simulink model "copper_solvent_extraction_model_simulink"  (R2021a)
settings: Solver=ode14x  StartTime=0.0  StopTime=simulation_time  FixedStep=step_time  RelTol=1e-3
undefined symbols (not defined in the file): C1_aq_ss, C1_el_ss, C1_org_ss, C2_aq_ss, C2_org_ss, C3_aq_ss, C3_org_ss, C4_org_ss, C_aq_max, C_org_max, cLE_ss, cPLS_ss, EXTERNAL_VARIABLES_STEADY_STATE, fLE_max, fLO_max, fPLSP_ss, fPLSS_ss, I_FB1, I_FB2, K_eq_ext, K_eq_str, K_ff_FF1, K_ff_FF2, K_ff_FF3, K_ff_FF4, K_mass_1, K_mass_2, K_mass_3, K_mass_4, Kb_FB1, Kb_FB2, Kc_FB1, Kc_FB2, LOWPASS_FILTER_TUNING, seed_c_BO, seed_c_LE, seed_c_LO, seed_c_PLS, seed_c_RaffP, seed_c_RaffS, seed_c_RE, seed_f_LE, seed_f_LO, seed_f_PLSP, seed_f_PLSS, sigma_c_BO, sigma_c_LE, sigma_c_LO, sigma_c_PLS, sigma_c_RaffP, sigma_c_RaffS, sigma_c_RE, sigma_f_LE, sigma_f_LO, sigma_f_PLSP, sigma_f_PLSS, step_time, t1, t2, t3 ... (+43)
libraries: cstblocks x4, pid_lib x2
(part 1 of 3)
settings Model: Creator=piete  LastModifiedBy=piete
settings DataIOCC: ReturnWorkspaceOutputsName=simulation_results

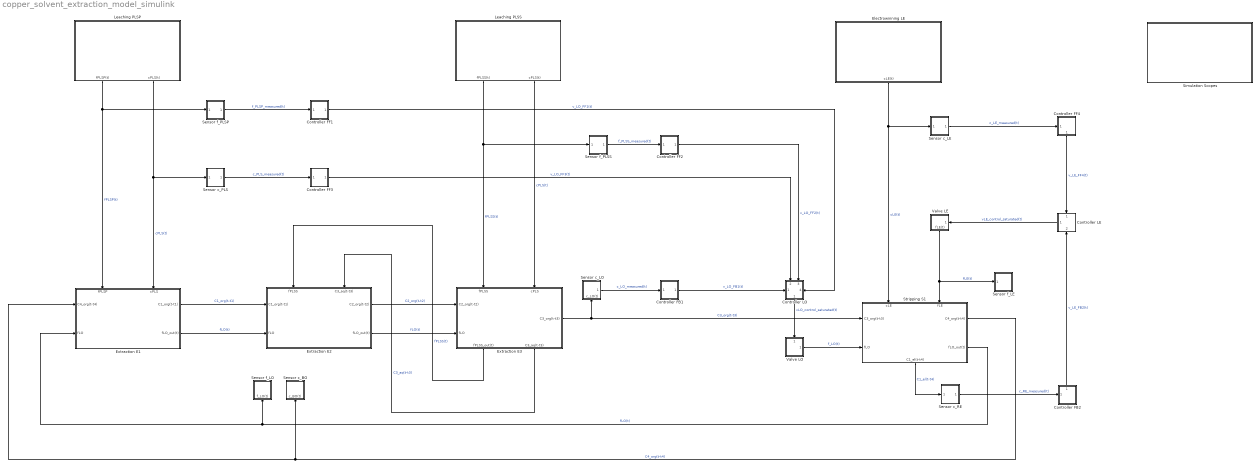
== system copper_solvent_extraction_model_simulink ==
  "                           Controller LO" : Subsystem
      settings: PortSchema="{\"entries\":[{\"content\":{\"sides\":[{\"content\":{\"connectorIds\":[\"In1\"]},\"type\":\"ConnectorPlacement.EquallySpacedRectSide\",\"uuid\":\"52743177-f082-4040-b095-38ff8f699919\"},{\"content\":{\"connectorIds\":[\"In4\"],\"side\":\"RIGHT\"},\"type\":\"ConnectorPlacement.EquallySpacedRectSide\",\"uuid\":\"070049ef-ea19-4899-84de-48e128addf57\"},{\"content\":{\"connectorIds\":[\"In2\",\"In3\"],\"side\":\"TOP\"},\"type\":\"ConnectorPlacement.EquallySpacedRectSide\",\"uuid\":\"35f470f2-3d73-4a31-9332-3265bce356f1\"},{\"content\":{\"connectorIds\":[\"Out1\"],\"side\":\"BOTTOM\"},\"type\":\"ConnectorPlacement.EquallySpacedRectSide\",\"uuid\":\"171e56ae-489a-47d3-90fa-98f8654578fe\"}]},\"type\":\"ConnectorPlacement.EquallySpacedConnector\",\"uuid\":\"0a01319a-d0cf-448a-a915-1b81fd6ea2a4\"}],\"packageUris\":[\"http://schema.mathworks.com/mf0/Connector/R2020b\"],\"version\":\"1.0\"}"
      mask Display: image('.\assets\simulink\controllers\c_LO_controller.png'); % Use "Edit Image" on toolstrip to change.
  Controller FB1 : Subsystem
      mask Display: image('.\assets\simulink\controllers\controller_FB1.png'); % Use "Edit Image" on toolstrip to change.
  Controller FB2 : Subsystem
      settings: PortSchema="{\"entries\":[{\"content\":{\"sides\":[{\"content\":{\"connectorIds\":[\"In1\"]},\"type\":\"ConnectorPlacement.EquallySpacedRectSide\",\"uuid\":\"549d450d-0da5-494d-9dce-c33c7378f634\"},{\"content\":{\"connectorIds\":[],\"side\":\"RIGHT\"},\"type\":\"ConnectorPlacement.EquallySpacedRectSide\",\"uuid\":\"cc4f927b-a34a-449e-b64f-caed187c260d\"},{\"content\":{\"connectorIds\":[\"Out1\"],\"side\":\"TOP\"},\"type\":\"ConnectorPlacement.EquallySpacedRectSide\",\"uuid\":\"b52d82b8-907a-4fce-9f5e-46f0b202510f\"}]},\"type\":\"ConnectorPlacement.EquallySpacedConnector\",\"uuid\":\"8987fc10-9638-4425-b9e3-d065bbee564b\"}],\"packageUris\":[\"http://schema.mathworks.com/mf0/Connector/R2020b\"],\"version\":\"1.0\"}"
      mask Display: image('.\assets\simulink\controllers\controller_FB2.png'); % Use "Edit Image" on toolstrip to change.
  Controller FF1 : Subsystem
      mask Display: image('.\assets\simulink\controllers\controller_FF1.png'); % Use "Edit Image" on toolstrip to change.
  Controller FF2 : Subsystem
      mask Display: image('.\assets\simulink\controllers\controller_FF2.png'); % Use "Edit Image" on toolstrip to change.
  Controller FF3 : Subsystem
      mask Display: image('.\assets\simulink\controllers\controller_FF3.png'); % Use "Edit Image" on toolstrip to change.
  Controller FF4 : Subsystem
      settings: PortSchema="{\"entries\":[{\"content\":{\"sides\":[{\"content\":{\"connectorIds\":[\"In1\"]},\"type\":\"ConnectorPlacement.EquallySpacedRectSide\",\"uuid\":\"309a0a3d-e30b-4a77-b5d2-c4b50080f33a\"},{\"content\":{\"connectorIds\":[],\"side\":\"RIGHT\"},\"type\":\"ConnectorPlacement.EquallySpacedRectSide\",\"uuid\":\"b344a8f7-ad8f-4273-abc7-1e7d20895348\"},{\"content\":{\"connectorIds\":[],\"side\":\"TOP\"},\"type\":\"ConnectorPlacement.EquallySpacedRectSide\",\"uuid\":\"47acaef9-06fd-4941-bd8f-4f44734e5892\"},{\"content\":{\"connectorIds\":[\"Out1\"],\"side\":\"BOTTOM\"},\"type\":\"ConnectorPlacement.EquallySpacedRectSide\",\"uuid\":\"0fe3c328-0dcb-42fe-b977-ff04426d3ff8\"}]},\"type\":\"ConnectorPlacement.EquallySpacedConnector\",\"uuid\":\"cf890694-841f-4aa2-8bc3-028381901d63\"}],\"packageUris\":[\"http://schema.mathworks.com/mf0/Connector/R2020b\"],\"version\":\"1.0\"}"
      mask Display: image('.\assets\simulink\controllers\controller_FF4.png'); % Use "Edit Image" on toolstrip to change.
  Controller LE : Subsystem
      settings: PortSchema="{\"entries\":[{\"content\":{\"sides\":[{\"content\":{\"connectorIds\":[]},\"type\":\"ConnectorPlacement.EquallySpacedRectSide\",\"uuid\":\"549d450d-0da5-494d-9dce-c33c7378f634\"},{\"content\":{\"connectorIds\":[\"Out1\"],\"side\":\"RIGHT\"},\"type\":\"ConnectorPlacement.EquallySpacedRectSide\",\"uuid\":\"cc4f927b-a34a-449e-b64f-caed187c260d\"},{\"content\":{\"connectorIds\":[\"In1\"],\"side\":\"TOP\"},\"type\":\"ConnectorPlacement.EquallySpacedRectSide\",\"uuid\":\"b52d82b8-907a-4fce-9f5e-46f0b202510f\"},{\"content\":{\"connectorIds\":[\"In2\"],\"side\":\"BOTTOM\"},\"type\":\"ConnectorPlacement.EquallySpacedRectSide\",\"uuid\":\"d43d3a57-d85d-4e24-871d-d5e185b00129\"}]},\"type\":\"ConnectorPlacement.EquallySpacedConnector\",\"uuid\":\"8987fc10-9638-4425-b9e3-d065bbee564b\"}],\"packageUris\":[\"http://schema.mathworks.com/mf0/Connector/R2020b\"],\"version\":\"1.0\"}"
      mask Display: image('.\assets\simulink\controllers\c_RE_controller.png'); % Use "Edit Image" on toolstrip to change.
  Electrowinning LE : Subsystem
      settings: PortSchema="{\"entries\":[{\"content\":{\"sides\":[{\"content\":{\"connectorIds\":[]},\"type\":\"ConnectorPlacement.EquallySpacedRectSide\",\"uuid\":\"d08e9f48-9437-4d33-afd1-67836a5fb6bd\"},{\"content\":{\"connectorIds\":[],\"side\":\"RIGHT\"},\"type\":\"ConnectorPlacement.EquallySpacedRectSide\",\"uuid\":\"a0c0d898-7ac9-474d-9070-540f9b51cc10\"},{\"content\":{\"connectorIds\":[],\"side\":\"TOP\"},\"type\":\"ConnectorPlacement.EquallySpacedRectSide\",\"uuid\":\"8a168008-9249-431e-9938-add887b6cc49\"},{\"content\":{\"connectorIds\":[\"Out1\"],\"side\":\"BOTTOM\"},\"type\":\"ConnectorPlacement.EquallySpacedRectSide\",\"uuid\":\"b6c2cc53-6d77-4314-bf25-d5a8095a8509\"}]},\"type\":\"ConnectorPlacement.EquallySpacedConnector\",\"uuid\":\"c94c7a5d-e9b9-4155-acb9-8888f4595dcb\"}],\"packageUris\":[\"http://schema.mathworks.com/mf0/Connector/R2020b\"],\"version\":\"1.0\"}"
      mask Display: image('.\assets\simulink\main_processes\LE.png'); % Use "Edit Image" on toolstrip to change.
  Extraction E1 : Subsystem
      settings: PortSchema="{\"entries\":[{\"content\":{\"sides\":[{\"content\":{\"connectorIds\":[\"In1\",\"In2\"]},\"type\":\"ConnectorPlacement.EquallySpacedRectSide\",\"uuid\":\"f32559ae-5e45-417b-8c50-adbeea9a29f4\"},{\"content\":{\"connectorIds\":[\"Out1\",\"Out2\"],\"side\":\"RIGHT\"},\"type\":\"ConnectorPlacement.EquallySpacedRectSide\",\"uuid\":\"22bc39ae-803b-4947-b021-a54bd767cf3b\"},{\"content\":{\"connectorIds\":[\"In3\",\"In4\"],\"side\":\"TOP\"},\"type\":\"ConnectorPlacement.EquallySpacedRectSide\",\"uuid\":\"d59dc34f-8db0-4177-a2fb-6760d02603f2\"}]},\"type\":\"ConnectorPlacement.EquallySpacedConnector\",\"uuid\":\"eadb17fe-3c9c-4f7d-9ae7-0fe299ce1ce3\"}],\"packageUris\":[\"http://schema.mathworks.com/mf0/Connector/R2020b\"],\"version\":\"1.0\"}"
      mask Display: image('.\assets\simulink\main_processes\E1.png'); % Use "Edit Image" on toolstrip to change.
  Extraction E2 : Subsystem
      settings: PortSchema="{\"entries\":[{\"content\":{\"sides\":[{\"content\":{\"connectorIds\":[\"In1\",\"In2\"]},\"type\":\"ConnectorPlacement.EquallySpacedRectSide\",\"uuid\":\"f32559ae-5e45-417b-8c50-adbeea9a29f4\"},{\"content\":{\"connectorIds\":[\"Out1\",\"Out2\"],\"side\":\"RIGHT\"},\"type\":\"ConnectorPlacement.EquallySpacedRectSide\",\"uuid\":\"22bc39ae-803b-4947-b021-a54bd767cf3b\"},{\"content\":{\"connectorIds\":[\"In3\",\"In4\"],\"side\":\"TOP\"},\"type\":\"ConnectorPlacement.EquallySpacedRectSide\",\"uuid\":\"d59dc34f-8db0-4177-a2fb-6760d02603f2\"}]},\"type\":\"ConnectorPlacement.EquallySpacedConnector\",\"uuid\":\"eadb17fe-3c9c-4f7d-9ae7-0fe299ce1ce3\"}],\"packageUris\":[\"http://schema.mathworks.com/mf0/Connector/R2020b\"],\"version\":\"1.0\"}"
      mask Display: image('.\assets\simulink\main_processes\E2.png'); % Use "Edit Image" on toolstrip to change.
  Extraction E3 : Subsystem
      settings: PortSchema="{\"entries\":[{\"content\":{\"sides\":[{\"content\":{\"connectorIds\":[\"In1\",\"In2\"]},\"type\":\"ConnectorPlacement.EquallySpacedRectSide\",\"uuid\":\"f32559ae-5e45-417b-8c50-adbeea9a29f4\"},{\"content\":{\"connectorIds\":[\"Out1\"],\"side\":\"RIGHT\"},\"type\":\"ConnectorPlacement.EquallySpacedRectSide\",\"uuid\":\"22bc39ae-803b-4947-b021-a54bd767cf3b\"},{\"content\":{\"connectorIds\":[\"In3\",\"In4\"],\"side\":\"TOP\"},\"type\":\"ConnectorPlacement.EquallySpacedRectSide\",\"uuid\":\"d59dc34f-8db0-4177-a2fb-6760d02603f2\"},{\"content\":{\"connectorIds\":[\"Out2\",\"Out3\"],\"side\":\"BOTTOM\"},\"type\":\"ConnectorPlacement.EquallySpacedRectSide\",\"uuid\":\"fbeb4835-7edf-4107-b431-1a8f0a3c5582\"}]},\"type\":\"ConnectorPlacement.EquallySpacedConnector\",\"uuid\":\"eadb17fe-3c9c-4f7d-9ae7-0fe299ce1ce3\"}],\"packageUris\":[\"http://schema.mathworks.com/mf0/Connector/R2020b\"],\"version\":\"1.0\"}"
      mask Display: image('.\assets\simulink\main_processes\E3.png'); % Use "Edit Image" on toolstrip to change.
  Leaching PLSP : Subsystem
      settings: PortSchema="{\"entries\":[{\"content\":{\"sides\":[{\"content\":{\"connectorIds\":[]},\"type\":\"ConnectorPlacement.EquallySpacedRectSide\",\"uuid\":\"350927fc-4dd2-494c-92db-8910e4459de4\"},{\"content\":{\"connectorIds\":[],\"side\":\"RIGHT\"},\"type\":\"ConnectorPlacement.EquallySpacedRectSide\",\"uuid\":\"54b31e5b-e75a-43e6-8723-66b6669f42f1\"},{\"content\":{\"connectorIds\":[],\"side\":\"TOP\"},\"type\":\"ConnectorPlacement.EquallySpacedRectSide\",\"uuid\":\"70d3a06c-9c50-446d-baab-5ad4a4ca1d21\"},{\"content\":{\"connectorIds\":[\"Out1\",\"Out2\"],\"side\":\"BOTTOM\"},\"type\":\"ConnectorPlacement.EquallySpacedRectSide\",\"uuid\":\"692c27e6-c427-4995-97d0-ac5f1bf9d541\"}]},\"type\":\"ConnectorPlacement.EquallySpacedConnector\",\"uuid\":\"478cabe5-44a5-4e19-b357-ea716b81ddf8\"}],\"packageUris\":[\"http://schema.mathworks.com/mf0/Connector/R2020b\"],\"version\":\"1.0\"}"
      mask Display: image('.\assets\simulink\main_processes\PLSP.png'); % Use "Edit Image" on toolstrip to change.
  Leaching PLSS : Subsystem
      settings: PortSchema="{\"entries\":[{\"content\":{\"sides\":[{\"content\":{\"connectorIds\":[]},\"type\":\"ConnectorPlacement.EquallySpacedRectSide\",\"uuid\":\"350927fc-4dd2-494c-92db-8910e4459de4\"},{\"content\":{\"connectorIds\":[],\"side\":\"RIGHT\"},\"type\":\"ConnectorPlacement.EquallySpacedRectSide\",\"uuid\":\"54b31e5b-e75a-43e6-8723-66b6669f42f1\"},{\"content\":{\"connectorIds\":[],\"side\":\"TOP\"},\"type\":\"ConnectorPlacement.EquallySpacedRectSide\",\"uuid\":\"70d3a06c-9c50-446d-baab-5ad4a4ca1d21\"},{\"content\":{\"connectorIds\":[\"Out1\",\"Out2\"],\"side\":\"BOTTOM\"},\"type\":\"ConnectorPlacement.EquallySpacedRectSide\",\"uuid\":\"692c27e6-c427-4995-97d0-ac5f1bf9d541\"}]},\"type\":\"ConnectorPlacement.EquallySpacedConnector\",\"uuid\":\"478cabe5-44a5-4e19-b357-ea716b81ddf8\"}],\"packageUris\":[\"http://schema.mathworks.com/mf0/Connector/R2020b\"],\"version\":\"1.0\"}"
      mask Display: image('.\assets\simulink\main_processes\PLSS.png'); % Use "Edit Image" on toolstrip to change.
  Sensor c_BO : Subsystem
      settings: PortSchema="{\"entries\":[{\"content\":{\"sides\":[{\"content\":{\"connectorIds\":[]},\"type\":\"ConnectorPlacement.EquallySpacedRectSide\",\"uuid\":\"6f225f75-77bd-4d33-9eaa-68626f4c93f8\"},{\"content\":{\"connectorIds\":[],\"side\":\"RIGHT\"},\"type\":\"ConnectorPlacement.EquallySpacedRectSide\",\"uuid\":\"fc49b7bf-677f-4e67-b426-d7f20682fd5b\"},{\"content\":{\"connectorIds\":[],\"side\":\"TOP\"},\"type\":\"ConnectorPlacement.EquallySpacedRectSide\",\"uuid\":\"0f66abcc-726d-4049-9a2a-f7387bb5b454\"},{\"content\":{\"connectorIds\":[\"In1\"],\"side\":\"BOTTOM\"},\"type\":\"ConnectorPlacement.EquallySpacedRectSide\",\"uuid\":\"02c1b306-9984-45d6-a119-b92d8916e7f3\"}]},\"type\":\"ConnectorPlacement.EquallySpacedConnector\",\"uuid\":\"3246ee4f-c332-4bf0-a096-1d04253049f7\"}],\"packageUris\":[\"http://schema.mathworks.com/mf0/Connector/R2020b\"],\"version\":\"1.0\"}"
      mask Display: image('.\assets\simulink\sensors\c_BO_sensor.png'); % Use "Edit Image" on toolstrip to change.
  Sensor c_LE : Subsystem
      mask Display: image('.\assets\simulink\sensors\c_LE_sensor.png'); % Use "Edit Image" on toolstrip to change.
  Sensor c_LO : Subsystem
      settings: PortSchema="{\"entries\":[{\"content\":{\"sides\":[{\"content\":{\"connectorIds\":[]},\"type\":\"ConnectorPlacement.EquallySpacedRectSide\",\"uuid\":\"6f225f75-77bd-4d33-9eaa-68626f4c93f8\"},{\"content\":{\"connectorIds\":[\"Out1\"],\"side\":\"RIGHT\"},\"type\":\"ConnectorPlacement.EquallySpacedRectSide\",\"uuid\":\"fc49b7bf-677f-4e67-b426-d7f20682fd5b\"},{\"content\":{\"connectorIds\":[],\"side\":\"TOP\"},\"type\":\"ConnectorPlacement.EquallySpacedRectSide\",\"uuid\":\"0f66abcc-726d-4049-9a2a-f7387bb5b454\"},{\"content\":{\"connectorIds\":[\"In1\"],\"side\":\"BOTTOM\"},\"type\":\"ConnectorPlacement.EquallySpacedRectSide\",\"uuid\":\"02c1b306-9984-45d6-a119-b92d8916e7f3\"}]},\"type\":\"ConnectorPlacement.EquallySpacedConnector\",\"uuid\":\"3246ee4f-c332-4bf0-a096-1d04253049f7\"}],\"packageUris\":[\"http://schema.mathworks.com/mf0/Connector/R2020b\"],\"version\":\"1.0\"}"
      mask Display: image('.\assets\simulink\sensors\c_LO_sensor.png'); % Use "Edit Image" on toolstrip to change.
  Sensor c_PLS : Subsystem
      mask Display: image('.\assets\simulink\sensors\c_PLS_sensor.png'); % Use "Edit Image" on toolstrip to change.
  Sensor c_RE : Subsystem
      mask Display: image('.\assets\simulink\sensors\c_RE_sensor.png'); % Use "Edit Image" on toolstrip to change.
  Sensor f_LE : Subsystem
      mask Display: image('.\assets\simulink\sensors\f_LE_sensor.png'); % Use "Edit Image" on toolstrip to change.
  Sensor f_LO : Subsystem
      settings: PortSchema="{\"entries\":[{\"content\":{\"sides\":[{\"content\":{\"connectorIds\":[]},\"type\":\"ConnectorPlacement.EquallySpacedRectSide\",\"uuid\":\"6f225f75-77bd-4d33-9eaa-68626f4c93f8\"},{\"content\":{\"connectorIds\":[],\"side\":\"RIGHT\"},\"type\":\"ConnectorPlacement.EquallySpacedRectSide\",\"uuid\":\"fc49b7bf-677f-4e67-b426-d7f20682fd5b\"},{\"content\":{\"connectorIds\":[],\"side\":\"TOP\"},\"type\":\"ConnectorPlacement.EquallySpacedRectSide\",\"uuid\":\"0f66abcc-726d-4049-9a2a-f7387bb5b454\"},{\"content\":{\"connectorIds\":[\"In1\"],\"side\":\"BOTTOM\"},\"type\":\"ConnectorPlacement.EquallySpacedRectSide\",\"uuid\":\"9f64ef61-0078-4c2b-bb4e-a94dd0622467\"}]},\"type\":\"ConnectorPlacement.EquallySpacedConnector\",\"uuid\":\"3246ee4f-c332-4bf0-a096-1d04253049f7\"}],\"packageUris\":[\"http://schema.mathworks.com/mf0/Connector/R2020b\"],\"version\":\"1.0\"}"
      mask Display: image('.\assets\simulink\sensors\f_LO_sensor.png'); % Use "Edit Image" on toolstrip to change.
  Sensor f_PLSP : Subsystem
      mask Display: image('.\assets\simulink\sensors\f_PLSP_sensor.png'); % Use "Edit Image" on toolstrip to change.
  Sensor f_PLSS : Subsystem
      mask Display: image('.\assets\simulink\sensors\f_PLSS_sensor.png'); % Use "Edit Image" on toolstrip to change.
  Simulation Scopes : Subsystem
      mask Display: image('.\assets\simulink\main_processes\scopes.png'); % Use "Edit Image" on toolstrip to change.
  Stripping S1 : Subsystem
      settings: PortSchema="{\"entries\":[{\"content\":{\"sides\":[{\"content\":{\"connectorIds\":[\"In1\",\"In2\"]},\"type\":\"ConnectorPlacement.EquallySpacedRectSide\",\"uuid\":\"edd2b024-3361-40c1-bf48-03bacc8752ae\"},{\"content\":{\"connectorIds\":[\"Out1\",\"Out2\"],\"side\":\"RIGHT\"},\"type\":\"ConnectorPlacement.EquallySpacedRectSide\",\"uuid\":\"73229bfa-5f94-46f0-92ab-46840454d51f\"},{\"content\":{\"connectorIds\":[\"In3\",\"In4\"],\"side\":\"TOP\"},\"type\":\"ConnectorPlacement.EquallySpacedRectSide\",\"uuid\":\"93068968-7869-4ed0-814c-03a88b1ad5d7\"},{\"content\":{\"connectorIds\":[\"Out3\"],\"side\":\"BOTTOM\"},\"type\":\"ConnectorPlacement.EquallySpacedRectSide\",\"uuid\":\"05c22c48-5ee0-4944-946b-00d184f09bd6\"}]},\"type\":\"ConnectorPlacement.EquallySpacedConnector\",\"uuid\":\"bf2ed9fb-a5ec-4d53-b289-eba7aea4b2cc\"}],\"packageUris\":[\"http://schema.mathworks.com/mf0/Connector/R2020b\"],\"version\":\"1.0\"}"
      mask Display: image('.\assets\simulink\main_processes\S1.png'); % Use "Edit Image" on toolstrip to change.
  Valve LE : Subsystem
      settings: PortSchema="{\"entries\":[{\"content\":{\"sides\":[{\"content\":{\"connectorIds\":[\"In1\"]},\"type\":\"ConnectorPlacement.EquallySpacedRectSide\",\"uuid\":\"06bfa01a-e663-49ea-90bb-597467147bdb\"},{\"content\":{\"connectorIds\":[],\"side\":\"RIGHT\"},\"type\":\"ConnectorPlacement.EquallySpacedRectSide\",\"uuid\":\"1b97bf0a-d157-483d-9143-b19205f93668\"},{\"content\":{\"connectorIds\":[],\"side\":\"TOP\"},\"type\":\"ConnectorPlacement.EquallySpacedRectSide\",\"uuid\":\"96bb4535-0a27-4f39-8065-f058199dbb07\"},{\"content\":{\"connectorIds\":[\"Out1\"],\"side\":\"BOTTOM\"},\"type\":\"ConnectorPlacement.EquallySpacedRectSide\",\"uuid\":\"185cf173-893e-45df-b22c-8330d77439f7\"}]},\"type\":\"ConnectorPlacement.EquallySpacedConnector\",\"uuid\":\"e8ce835b-977e-44e0-89a4-4c36a3371ef1\"}],\"packageUris\":[\"http://schema.mathworks.com/mf0/Connector/R2020b\"],\"version\":\"1.0\"}"
      mask Display: image('.\assets\simulink\valves\Valve_LE.png'); % Use "Edit Image" on toolstrip to change.
  Valve LO : Subsystem
      settings: PortSchema="{\"entries\":[{\"content\":{\"sides\":[{\"content\":{\"connectorIds\":[]},\"type\":\"ConnectorPlacement.EquallySpacedRectSide\",\"uuid\":\"6fe3adae-c1d5-49c5-9f64-d9648a674ed6\"},{\"content\":{\"connectorIds\":[\"Out1\"],\"side\":\"RIGHT\"},\"type\":\"ConnectorPlacement.EquallySpacedRectSide\",\"uuid\":\"5144e458-c494-45ed-932f-5f38aa1be950\"},{\"content\":{\"connectorIds\":[\"In1\"],\"side\":\"TOP\"},\"type\":\"ConnectorPlacement.EquallySpacedRectSide\",\"uuid\":\"1ebd3b40-fd5b-41a9-a787-94161d466247\"}]},\"type\":\"ConnectorPlacement.EquallySpacedConnector\",\"uuid\":\"aaf376a4-907c-4b9b-913e-19faf97da0c8\"}],\"packageUris\":[\"http://schema.mathworks.com/mf0/Connector/R2020b\"],\"version\":\"1.0\"}"
      mask Display: image('.\assets\simulink\valves\Valve_LO.png'); % Use "Edit Image" on toolstrip to change.
  wires:
  Leaching PLSP/1(fPLSP(t)) -> Extraction E1/3(fPLSP), Sensor f_PLSP/1(f_PLSP(t))  "fPLSP(t)"
  Leaching PLSP/2(cPLS(t)) -> Extraction E1/4(cPLS), Sensor c_PLS/1(c_PLS(t))  "cPLS(t)"
  Electrowinning LE/1(cLE(t)) -> Stripping S1/3(cLE), Sensor c_LE/1(c_LE(t))  "cLE(t)"
  Valve LO/1(f_LO(t)) -> Stripping S1/2(fLO)  "f_LO(t)"
  Valve LE/1(fLE(t)) -> Sensor f_LE/1(f_LE(t)), Stripping S1/4(fLE)  "fLE(t)"
  Extraction E1/1(C1_org(t-t1)) -> Extraction E2/1(C1_org(t-t1))  "C1_org(t-t1)"
  Extraction E2/1(C2_org(t-t2)) -> Extraction E3/1(C2_org(t-t2))  "C2_org(t-t2)"
  Extraction E3/1(C3_org(t-t3)) -> Stripping S1/1(C3_org(t-t3)), Sensor c_LO/1(c_LO(t))  "C3_org(t-t3)"
  Stripping S1/3(C1_el(t-t4)) -> Sensor c_RE/1(c_RE(t))  "C1_el(t-t4)"
  Leaching PLSS/1(fPLSS(t)) -> Extraction E3/3(fPLSS), Sensor f_PLSS/1(f_PLSS(t))  "fPLSS(t)"
  Leaching PLSS/2(cPLS(t)) -> Extraction E3/4(cPLS)  "cPLS(t)"
  Extraction E1/2(fLO_out(t)) -> Extraction E2/2(fLO)  "fLO(t)"
  Extraction E2/2(fLO_out(t)) -> Extraction E3/2(fLO)  "fLO(t)"
  Stripping S1/2(fLO_out(t)) -> Sensor f_LO/1(f_LO(t)), Extraction E1/2(fLO)  "fLO(t)"
  Stripping S1/1(C4_org(t-t4)) -> Sensor c_BO/1(c_BO(t)), Extraction E1/1(C4_org(t-t4))  "C4_org(t-t4)"
  "                           Controller LO"/1(vLO_control_saturated(t)) -> Valve LO/1(vLO_control_saturated(t))  "vLO_control_saturated(t)"
  Controller LE/1(vLE_control_saturated(t)) -> Valve LE/1(vLE_control_saturated(t))  "vLE_control_saturated(t)"
  Extraction E3/2(fPLSS_out(t)) -> Extraction E2/3(fPLSS)  "fPLSS(t)"
  Extraction E3/3(C3_aq(t-t3)) -> Extraction E2/4(C3_aq(t-t3))  "C3_aq(t-t3)"
  Sensor c_LO/1(c_LO_measured(t)) -> Controller FB1/1(c_LO_measured(t))  "c_LO_measured(t)"
  Controller FB1/1(v_LO_FB1(t)) -> "                           Controller LO"/1(v_LO_FB1(t))  "v_LO_FB1(t)"
  Sensor c_RE/1(c_RE_measured(t)) -> Controller FB2/1(c_RE_measured(t))  "c_RE_measured(t)"
  Controller FB2/1(v_LE_FB2(t)) -> Controller LE/2(v_LE_FB2(t))  "v_LE_FB2(t)"
  Sensor f_PLSP/1(f_PLSP_measured(t)) -> Controller FF1/1(f_PLSP_measured(t))  "f_PLSP_measured(t)"
  Controller FF1/1(v_LO_FF1(t)) -> "                           Controller LO"/4(v_LO_FF1(t))  "v_LO_FF1(t)"
  Sensor f_PLSS/1(f_PLSS_measured(t)) -> Controller FF2/1(f_PLSS_measured(t))  "f_PLSS_measured(t)"
  Controller FF2/1(v_LO_FF2(t)) -> "                           Controller LO"/3("v_LO_FF2(t) ")  "v_LO_FF2(t)"
  Sensor c_PLS/1(c_PLS_measured(t)) -> Controller FF3/1(c_PLS_measured(t))  "c_PLS_measured(t)"
  Controller FF3/1(v_LO_FF3(t)) -> "                           Controller LO"/2(v_LO_FF3(t))  "v_LO_FF3(t)"
  Controller FF4/1(v_LE_FF4(t)) -> Controller LE/1(v_LE_FF4(t))  "v_LE_FF4(t)"
  Sensor c_LE/1(c_LE_measured(t)) -> Controller FF4/1(c_LE_measured(t))  "c_LE_measured(t)"

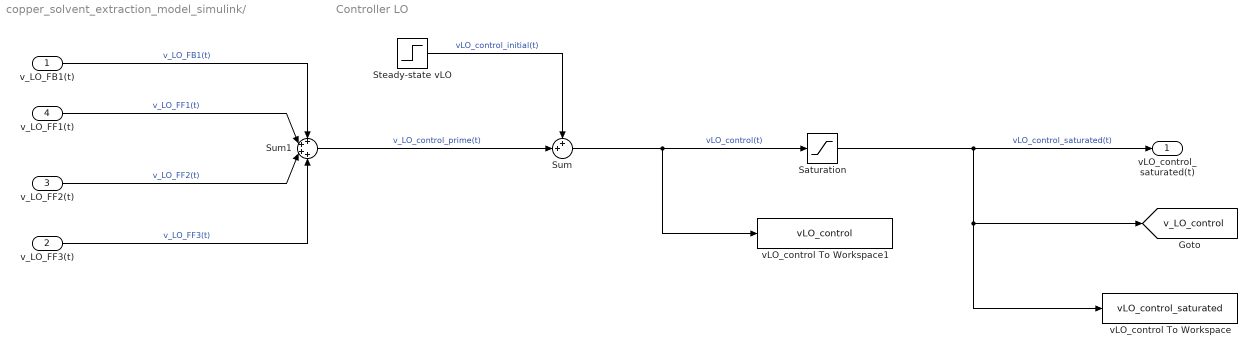
== system copper_solvent_extraction_model_simulink/                           Controller LO ==
  v_LO_FB1(t) : Inport
  v_LO_FF3(t) : Inport  Port=2
  "v_LO_FF2(t) " : Inport  Port=3
  v_LO_FF1(t) : Inport  Port=4
  Saturation : Saturate  UpperLimit=1  LowerLimit=0
  Steady-state vLO : Step  Time=0  Before=vLO_ss  After=vLO_ss  SampleTime=0
  Sum : Sum  Inputs=++|
  Sum1 : Sum  Inputs=++++
  vLO_control To Workspace : ToWorkspace  VariableName=vLO_control_saturated  SaveFormat=Timeseries  SampleTime=-1
  vLO_control To Workspace1 : ToWorkspace  VariableName=vLO_control  SaveFormat=Timeseries  SampleTime=-1
  vLO_control_saturated(t) : Outport
  tag scope: v_LO_control=global
  wires:
  Saturation/1 -> [v_LO_control], vLO_control To Workspace/1, vLO_control_saturated(t)/1  "vLO_control_saturated(t)"
  Steady-state vLO/1 -> Sum/1  "vLO_control_initial(t)"
  Sum1/1 -> Sum/2  "v_LO_control_prime(t)"
  Sum/1 -> Saturation/1, vLO_control To Workspace1/1  "vLO_control(t)"
  v_LO_FB1(t)/1 -> Sum1/1  "v_LO_FB1(t)"
  v_LO_FF1(t)/1 -> Sum1/2  "v_LO_FF1(t)"
  "v_LO_FF2(t) "/1 -> Sum1/3  "v_LO_FF2(t)"
  v_LO_FF3(t)/1 -> Sum1/4  "v_LO_FF3(t)"

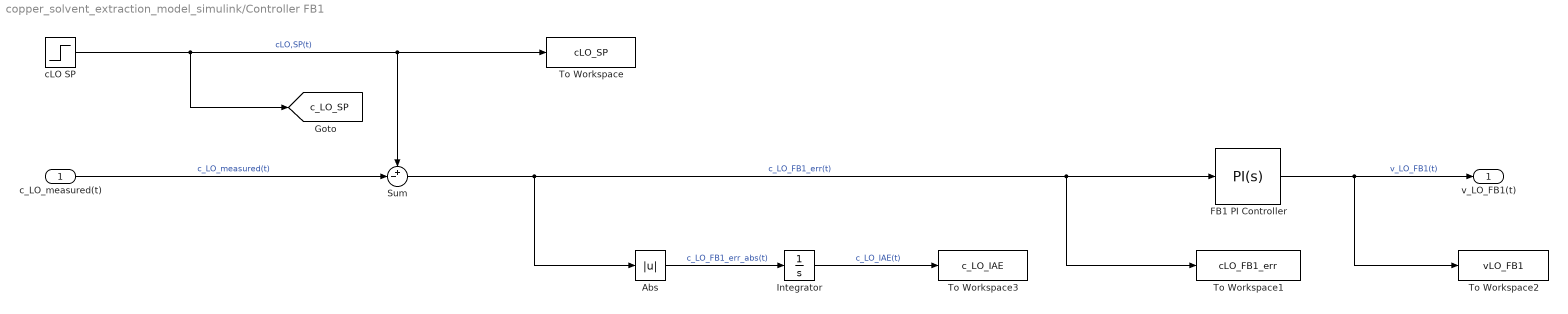
== system copper_solvent_extraction_model_simulink/Controller FB1 ==
  c_LO_measured(t) : Inport
  Abs : Abs
  FB1 PI Controller : pid_lib/PID Controller  Controller=PI  Form=Ideal  TimeDomain=Continuous-time  UseExternalTs=off  SampleTime=-1  IntegratorMethod=Forward Euler  FilterMethod=Forward Euler  ControllerParametersSource=internal  P=Kc_FB1  I=I_FB1  D=0  UseFilter=on  N=100  TunerSelectOption=Transfer Function Based (PID Tuner App)  InitialConditionSource=internal  InitialConditionForIntegrator=0  InitialConditionForFilter=0  DifferentiatorICPrevScaledInput=0  ExternalReset=none  TrackingMode=off  Kt=1  LimitOutput=on  SatLimitsSource=internal  UpperSaturationLimit=1-vLO_ss  LowerSaturationLimit=-vLO_ss  LinearizeAsGain=on  AntiWindupMode=back-calculation  Kb=Kb_FB1  POutMin=[]  POutMax=[]  IOutMin=[]  IOutMax=[]  DOutMin=[]  DOutMax=[]  NOutMin=[]  NOutMax=[]  SumOutMin=[]  SumOutMax=[]  SaturationOutMin=[]  SaturationOutMax=[]  PParamMin=[]  PParamMax=[]  IParamMin=[]  IParamMax=[]  DParamMin=[]  DParamMax=[]  NParamMin=[]  NParamMax=[]  KbParamMin=[]  KbParamMax=[]  KtParamMin=[]  KtParamMax=[]  KbOutMin=[]  KbOutMax=[]  KtOutMin=[]  KtOutMax=[]  IntegratorOutMin=[]  IntegratorOutMax=[]  FilterOutMin=[]  FilterOutMax=[]  SumI1OutMin=[]  SumI1OutMax=[]  SumI2OutMin=[]  SumI2OutMax=[]  SumI3OutMin=[]  SumI3OutMax=[]  SumI4OutMin=[]  SumI4OutMax=[]  SumDOutMin=[]  SumDOutMax=[]  DifferentiatorOutMin=[]  DifferentiatorOutMax=[]  FilterDiffOutCoefMin=[]  FilterDiffOutCoefMax=[]  ReciprocalOutMin=[]  ReciprocalOutMax=[]  SumDenOutMin=[]  SumDenOutMax=[]  SumNumOutMin=[]  SumNumOutMax=[]  DivideOutMin=[]  DivideOutMax=[]  UdiffTsProdOutMin=[]  UdiffTsProdOutMax=[]  NTsProdOutMin=[]  NTsProdOutMax=[]  UintegralTsProdOutMin=[]  UintegralTsProdOutMax=[]  UngainTsProdOutMin=[]  UngainTsProdOutMax=[]  IntegratorContinuousStateAttributes=''  IntegratorStateMustResolveToSignalObject=off  IntegratorRTWStateStorageClass=Auto  FilterContinuousStateAttributes=''  FilterStateMustResolveToSignalObject=off  FilterRTWStateStorageClass=Auto  ParallelPVariant=Passthrough  IdealPVariant=InternalParameters  IVariant=InternalParameters  DVariant=Disabled  IntegratorVariant=Continuous  SatVariant=Enabled  AWVariant=BackCalculation  PCopyVariant=Disabled  TRVariant=Disabled  FdbkBlocksVariant=Forward  IdealPFdbkVariant=Disabled  SatFdbkVariant=Disabled  DerivativeFilterVariant=Disabled  NVariant=Disabled  NCopyVariant=Disabled_SignalSpec  FilterICVariant=Disabled  IntegratorICVariant=InternalICs  ExternalResetVariant=Disabled  TRSumVariant=Passthrough  SumFdbkVariant=Disabled  SumVariant=Sum_PI  TsampFilterVariant=InternalTs  TsampNgainVariant=Passthrough  TsampIntegralVariant=Passthrough  ExternalSaturationOutDataTypeStr=Inherit: Same as second input
  Integrator : Integrator
  Sum : Sum  Inputs=+-|
  To Workspace : ToWorkspace  VariableName=cLO_SP  SaveFormat=Timeseries  SampleTime=-1
  To Workspace1 : ToWorkspace  VariableName=cLO_FB1_err  SaveFormat=Timeseries  SampleTime=-1
  To Workspace2 : ToWorkspace  VariableName=vLO_FB1  SaveFormat=Timeseries  SampleTime=-1
  To Workspace3 : ToWorkspace  VariableName=c_LO_IAE  SaveFormat=Timeseries  SampleTime=-1
  cLO SP : Step  Time=0  Before=C3_org_ss  After=C3_org_ss  SampleTime=0
  v_LO_FB1(t) : Outport
  tag scope: c_LO_SP=global
  wires:
  c_LO_measured(t)/1 -> Sum/2  "c_LO_measured(t)"
  cLO SP/1 -> [c_LO_SP], Sum/1, To Workspace/1  "cLO,SP(t)"
  Sum/1 -> FB1 PI Controller/1, To Workspace1/1, Abs/1  "c_LO_FB1_err(t)"
  FB1 PI Controller/1 -> To Workspace2/1, v_LO_FB1(t)/1  "v_LO_FB1(t)"
  Abs/1 -> Integrator/1  "c_LO_FB1_err_abs(t)"
  Integrator/1 -> To Workspace3/1  "c_LO_IAE(t)"

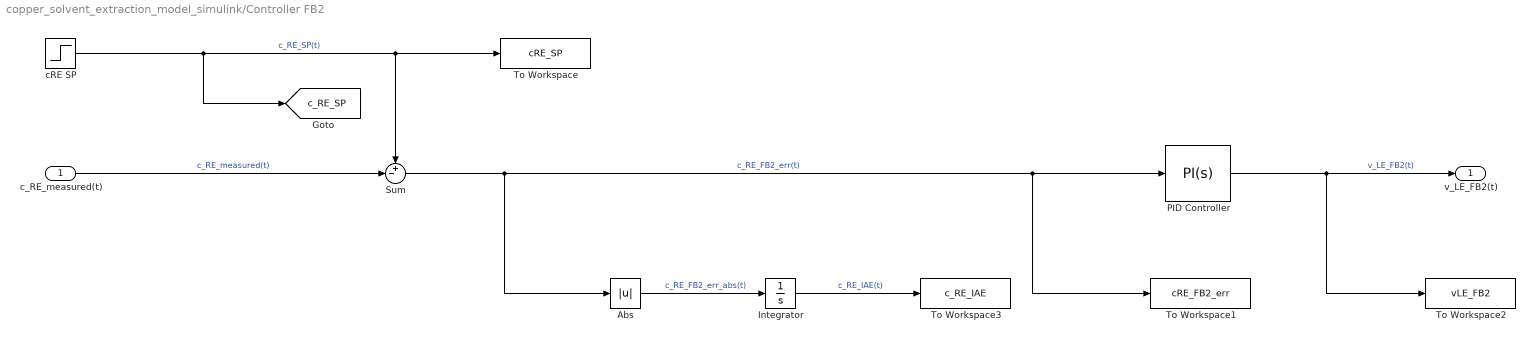
== system copper_solvent_extraction_model_simulink/Controller FB2 ==
  c_RE_measured(t) : Inport
  Abs : Abs
  Integrator : Integrator
  PID Controller : pid_lib/PID Controller  Controller=PI  Form=Ideal  TimeDomain=Continuous-time  UseExternalTs=off  SampleTime=-1  IntegratorMethod=Forward Euler  FilterMethod=Forward Euler  ControllerParametersSource=internal  P=Kc_FB2  I=I_FB2  D=0  UseFilter=on  N=100  TunerSelectOption=Transfer Function Based (PID Tuner App)  InitialConditionSource=internal  InitialConditionForIntegrator=0  InitialConditionForFilter=0  DifferentiatorICPrevScaledInput=0  ExternalReset=none  TrackingMode=off  Kt=1  LimitOutput=on  SatLimitsSource=internal  UpperSaturationLimit=1-vLE_ss  LowerSaturationLimit=-vLE_ss  LinearizeAsGain=on  AntiWindupMode=back-calculation  Kb=Kb_FB2  POutMin=[]  POutMax=[]  IOutMin=[]  IOutMax=[]  DOutMin=[]  DOutMax=[]  NOutMin=[]  NOutMax=[]  SumOutMin=[]  SumOutMax=[]  SaturationOutMin=[]  SaturationOutMax=[]  PParamMin=[]  PParamMax=[]  IParamMin=[]  IParamMax=[]  DParamMin=[]  DParamMax=[]  NParamMin=[]  NParamMax=[]  KbParamMin=[]  KbParamMax=[]  KtParamMin=[]  KtParamMax=[]  KbOutMin=[]  KbOutMax=[]  KtOutMin=[]  KtOutMax=[]  IntegratorOutMin=[]  IntegratorOutMax=[]  FilterOutMin=[]  FilterOutMax=[]  SumI1OutMin=[]  SumI1OutMax=[]  SumI2OutMin=[]  SumI2OutMax=[]  SumI3OutMin=[]  SumI3OutMax=[]  SumI4OutMin=[]  SumI4OutMax=[]  SumDOutMin=[]  SumDOutMax=[]  DifferentiatorOutMin=[]  DifferentiatorOutMax=[]  FilterDiffOutCoefMin=[]  FilterDiffOutCoefMax=[]  ReciprocalOutMin=[]  ReciprocalOutMax=[]  SumDenOutMin=[]  SumDenOutMax=[]  SumNumOutMin=[]  SumNumOutMax=[]  DivideOutMin=[]  DivideOutMax=[]  UdiffTsProdOutMin=[]  UdiffTsProdOutMax=[]  NTsProdOutMin=[]  NTsProdOutMax=[]  UintegralTsProdOutMin=[]  UintegralTsProdOutMax=[]  UngainTsProdOutMin=[]  UngainTsProdOutMax=[]  IntegratorContinuousStateAttributes=''  IntegratorStateMustResolveToSignalObject=off  IntegratorRTWStateStorageClass=Auto  FilterContinuousStateAttributes=''  FilterStateMustResolveToSignalObject=off  FilterRTWStateStorageClass=Auto  ParallelPVariant=Passthrough  IdealPVariant=InternalParameters  IVariant=InternalParameters  DVariant=Disabled  IntegratorVariant=Continuous  SatVariant=Enabled  AWVariant=BackCalculation  PCopyVariant=Disabled  TRVariant=Disabled  FdbkBlocksVariant=Forward  IdealPFdbkVariant=Disabled  SatFdbkVariant=Disabled  DerivativeFilterVariant=Disabled  NVariant=Disabled  NCopyVariant=Disabled_SignalSpec  FilterICVariant=Disabled  IntegratorICVariant=InternalICs  ExternalResetVariant=Disabled  TRSumVariant=Passthrough  SumFdbkVariant=Disabled  SumVariant=Sum_PI  TsampFilterVariant=InternalTs  TsampNgainVariant=Passthrough  TsampIntegralVariant=Passthrough  ExternalSaturationOutDataTypeStr=Inherit: Same as second input
  Sum : Sum  Inputs=+-|
  To Workspace : ToWorkspace  VariableName=cRE_SP  SaveFormat=Timeseries  SampleTime=-1
  To Workspace1 : ToWorkspace  VariableName=cRE_FB2_err  SaveFormat=Timeseries  SampleTime=-1
  To Workspace2 : ToWorkspace  VariableName=vLE_FB2  SaveFormat=Timeseries  SampleTime=-1
  To Workspace3 : ToWorkspace  VariableName=c_RE_IAE  SaveFormat=Timeseries  SampleTime=-1
  cRE SP : Step  Time=0  Before=C1_el_ss  After=C1_el_ss  SampleTime=0
  v_LE_FB2(t) : Outport
  tag scope: c_RE_SP=global
  wires:
  c_RE_measured(t)/1 -> Sum/2  "c_RE_measured(t)"
  cRE SP/1 -> [c_RE_SP], To Workspace/1, Sum/1  "c_RE_SP(t)"
  Sum/1 -> Abs/1, PID Controller/1, To Workspace1/1  "c_RE_FB2_err(t)"
  PID Controller/1 -> To Workspace2/1, v_LE_FB2(t)/1  "v_LE_FB2(t)"
  Integrator/1 -> To Workspace3/1  "c_RE_IAE(t)"
  Abs/1 -> Integrator/1  "c_RE_FB2_err_abs(t)"

== system copper_solvent_extraction_model_simulink/Controller FF1 ==
  f_PLSP_measured(t) : Inport
  Sum : Sum  Inputs=-+|
  To Workspace : ToWorkspace  VariableName=vLO_FF1  SaveFormat=Timeseries  SampleTime=-1
  Transfer Fcn : TransferFcn  Numerator=[K_ff_FF1*T_ld_FF1 K_ff_FF1*1]  Denominator=[T_lg_FF1 1]
  Transport Delay : TransportDelay  DelayTime=theta_ff_FF1
  f_PLSP_ss : Step  Time=0  Before=fPLSP_ss  After=fPLSP_ss  SampleTime=0
  v_LO_FF1(t) : Outport
  wires:
  Sum/1 -> Transfer Fcn/1  "f_PLSP_measured_prime(t)"
  Transport Delay/1 -> To Workspace/1, v_LO_FF1(t)/1  "v_LO_FF1(t)"
  Transfer Fcn/1 -> Transport Delay/1  "v_LO_FF1_pre_delay(t)"
  f_PLSP_measured(t)/1 -> Sum/2  "f_PLSP_measured(t)"
  f_PLSP_ss/1 -> Sum/1  "f_PLSP_ss"

== system copper_solvent_extraction_model_simulink/Controller FF2 ==
  f_PLSS_measured(t) : Inport
  Sum : Sum  Inputs=-+|
  To Workspace : ToWorkspace  VariableName=vLO_FF2  SaveFormat=Timeseries  SampleTime=-1
  Transfer Fcn : TransferFcn  Numerator=[K_ff_FF2*T_ld_FF2 K_ff_FF2*1]  Denominator=[T_lg_FF2 1]
  Transport Delay : TransportDelay  DelayTime=theta_ff_FF2
  f_PLSS_ss : Step  Time=0  Before=fPLSS_ss  After=fPLSS_ss  SampleTime=0
  v_LO_FF2(t) : Outport
  wires:
  Sum/1 -> Transfer Fcn/1  "f_PLSS_measured_prime(t)"
  Transport Delay/1 -> To Workspace/1, v_LO_FF2(t)/1  "v_LO_FF2(t)"
  Transfer Fcn/1 -> Transport Delay/1  "v_LO_FF2_pre_delay(t)"
  f_PLSS_measured(t)/1 -> Sum/2  "f_PLSS_measured(t)"
  f_PLSS_ss/1 -> Sum/1  "f_PLSS_ss"

== system copper_solvent_extraction_model_simulink/Controller FF3 ==
  c_PLS_measured(t) : Inport
  Sum : Sum  Inputs=-+|
  To Workspace : ToWorkspace  VariableName=vLO_FF3  SaveFormat=Timeseries  SampleTime=-1
  Transfer Fcn : TransferFcn  Numerator=[K_ff_FF3*T_ld_FF3 K_ff_FF3*1]  Denominator=[T_lg_FF3 1]
  Transport Delay : TransportDelay  DelayTime=theta_ff_FF3
  c_PLS_ss : Step  Time=0  Before=cPLS_ss  After=cPLS_ss  SampleTime=0
  v_LO_FF3(t) : Outport
  wires:
  Sum/1 -> Transfer Fcn/1  "c_PLS_measured_prime(t)"
  Transport Delay/1 -> To Workspace/1, v_LO_FF3(t)/1  "v_LO_FF3(t)"
  Transfer Fcn/1 -> Transport Delay/1  "v_LO_FF3_pre_delay(t)"
  c_PLS_measured(t)/1 -> Sum/2  "c_PLS_measured(t)"
  c_PLS_ss/1 -> Sum/1  "c_PLS_ss"

== system copper_solvent_extraction_model_simulink/Controller FF4 ==
  c_LE_measured(t) : Inport
  Sum : Sum  Inputs=-+|
  To Workspace : ToWorkspace  VariableName=vLE_FF4  SaveFormat=Timeseries  SampleTime=-1
  Transfer Fcn : TransferFcn  Numerator=[K_ff_FF4*T_ld_FF4 K_ff_FF4*1]  Denominator=[T_lg_FF4 1]
  Transport Delay : TransportDelay  DelayTime=theta_ff_FF4
  c_LE_ss : Step  Time=0  Before=cLE_ss  After=cLE_ss  SampleTime=0
  v_LE_FF4(t) : Outport
  wires:
  Sum/1 -> Transfer Fcn/1  "c_LE_measured_prime(t)"
  Transport Delay/1 -> To Workspace/1, v_LE_FF4(t)/1  "v_LE_FF4(t)"
  Transfer Fcn/1 -> Transport Delay/1  "v_LE_FF4_pre_delay(t)"
  c_LE_measured(t)/1 -> Sum/2  "c_LE_measured(t)"
  c_LE_ss/1 -> Sum/1  "c_LE_ss"

== system copper_solvent_extraction_model_simulink/Controller LE ==
  v_LE_FF4(t) : Inport
  v_LE_FB2(t) : Inport  Port=2
  Saturation : Saturate  UpperLimit=1  LowerLimit=0
  Steady-state vLE : Step  Time=0  Before=vLE_ss  After=vLE_ss  SampleTime=0
  Sum : Sum  Inputs=++|
  Sum1 : Sum  Inputs=+|+
  To Workspace : ToWorkspace  VariableName=vLE_control_saturated  SaveFormat=Timeseries  SampleTime=-1
  vLE_control To Workspace : ToWorkspace  VariableName=vLE_control  SaveFormat=Timeseries  SampleTime=-1
  vLE_control_saturated(t) : Outport
  tag scope: v_LE_control=global
  wires:
  Sum/1 -> Saturation/1, vLE_control To Workspace/1  "vLE_control(t)"
  Saturation/1 -> [v_LE_control], To Workspace/1, vLE_control_saturated(t)/1  "vLE_control_Saturated(t)"
  Sum1/1 -> Sum/2  "v_LE_control_prime(t)"
  Steady-state vLE/1 -> Sum/1  "vLE_control_initial(t)"
  v_LE_FB2(t)/1 -> Sum1/1  "v_LE_FB2(t)"
  v_LE_FF4(t)/1 -> Sum1/2  "v_LE_FF4(t)"

== system copper_solvent_extraction_model_simulink/Electrowinning LE ==
  Constant1 : Constant  Value=EXTERNAL_VARIABLES_STEADY_STATE
  From Workspace : FromWorkspace  VariableName=c_LE_timeseries
  Switch1 : Switch  Criteria=u2 ~= 0
  cLE : Step  Time=0  Before=cLE_ss  After=cLE_ss  SampleTime=0
  cLE To Workspace : ToWorkspace  VariableName=cLE  SaveFormat=Timeseries  SampleTime=-1
  cLE(t) : Outport
  wires:
  Switch1/1 -> cLE To Workspace/1, cLE(t)/1  "cLE(t)"
  Constant1/1 -> Switch1/2  "is_steady_state"
  cLE/1 -> Switch1/1  "cLE_steady_state(t)"
  From Workspace/1 -> Switch1/3  "cLE_non_steady_state(t)"

== system copper_solvent_extraction_model_simulink/Extraction E1 ==
  C4_org(t-t4) : Inport
  fLO : Inport  Port=2
  fPLSP : Inport  Port=3
  cPLS : Inport  Port=4
  Mixer E1 : Subsystem
      mask Display: image('.\assets\simulink\mixers_and_setlers\E1_mixer.png'); % Use "Edit Image" on toolstrip to change.
  Sensor c_RaffP : Subsystem
      mask Display: image('.\assets\simulink\sensors\c_RaffP_sensor.png'); % Use "Edit Image" on toolstrip to change.
  Settler E1 : Subsystem
      mask Display: image('.\assets\simulink\mixers_and_setlers\E1_settler.png'); % Use "Edit Image" on toolstrip to change.
  C1_org(t-t1) : Outport
  fLO_out(t) : Outport  Port=2
  wires:
  fLO/1 -> Mixer E1/3(fLO), fLO_out(t)/1  "fLO(t)"
  Mixer E1/2(C1_aq(t)) -> Settler E1/2(C1_aq(t))  "C1_aq(t)"
  cPLS/1 -> Mixer E1/2(cPLS)  "cPLS(t)"
  Mixer E1/1(C1_org(t)) -> Settler E1/1(C1_org(t))  "C1_org(t)"
  Settler E1/1(C1_org(t-t1)) -> C1_org(t-t1)/1  "C1_org(t-t1)"
  fPLSP/1 -> Mixer E1/1(fPLSP)  "fPLSP(t)"
  C4_org(t-t4)/1 -> Mixer E1/4(C4_org(t-t4))  "C4_org(t-t4)"
  Settler E1/2(C1_aq(t-t1)) -> Sensor c_RaffP/1(c_RaffP(t))  "C1_aq(t-t1)"

== system copper_solvent_extraction_model_simulink/Extraction E2 ==
  C1_org(t-t1) : Inport
  fLO : Inport  Port=2
  fPLSS : Inport  Port=3
  C3_aq(t-t3) : Inport  Port=4
  Mixer E2 : Subsystem
      mask Display: image('.\assets\simulink\mixers_and_setlers\E2_mixer.png'); % Use "Edit Image" on toolstrip to change.
  Sensor c_RaffS : Subsystem
      mask Display: image('.\assets\simulink\sensors\c_RaffS_sensor.png'); % Use "Edit Image" on toolstrip to change.
  Settler E2 : Subsystem
      mask Display: image('.\assets\simulink\mixers_and_setlers\E2_settler.png'); % Use "Edit Image" on toolstrip to change.
  C2_org(t-t2) : Outport
  fLO_out(t) : Outport  Port=2
  wires:
  C3_aq(t-t3)/1 -> Mixer E2/2(C3_aq(t-t3))  "C3_aq(t-t3)"
  Mixer E2/1(C2_org(t)) -> Settler E2/1(C2_org(t))  "C2_org(t)"
  Mixer E2/2(C2_aq(t)) -> Settler E2/2(C2_aq(t))  "C2_aq(t)"
  Settler E2/1(C2_org(t-t2)) -> C2_org(t-t2)/1  "C2_org(t-t2)"
  fLO/1 -> fLO_out(t)/1, Mixer E2/3(fLO)  "fLO(t)"
  C1_org(t-t1)/1 -> Mixer E2/4(C1_org(t-t1))  "C1_org(t-t1)"
  fPLSS/1 -> Mixer E2/1(fPLSS)  "fPLSS(t)"
  Settler E2/2(C2_aq(t-t2)) -> Sensor c_RaffS/1(c_RaffS(t))  "C2_aq(t-t2)"

== system copper_solvent_extraction_model_simulink/Extraction E3 ==
  C2_org(t-t2) : Inport
  fLO : Inport  Port=2
  fPLSS : Inport  Port=3
  cPLS : Inport  Port=4
  Mixer E3 : Subsystem
      mask Display: image('.\assets\simulink\mixers_and_setlers\E3_mixer.png'); % Use "Edit Image" on toolstrip to change.
  Settler E3 : Subsystem
      mask Display: image('.\assets\simulink\mixers_and_setlers\E3_settler.png'); % Use "Edit Image" on toolstrip to change.
  C3_org(t-t3) : Outport
  fPLSS_out(t) : Outport  Port=2
  C3_aq(t-t3) : Outport  Port=3
  wires:
  C2_org(t-t2)/1 -> Mixer E3/4(C2_org(t-t2))  "C2_org(t-t2)"
  cPLS/1 -> Mixer E3/2(cPLS)  "cPLS(t)"
  Mixer E3/1(C3_org(t)) -> Settler E3/1(C3_org(t))  "C3_org(t)"
  fPLSS/1 -> fPLSS_out(t)/1, Mixer E3/1(fPLSS)  "fPLSS(t)"
  Mixer E3/2(C3_aq(t)) -> Settler E3/2(C3_aq(t))  "C3_aq(t)"
  Settler E3/1(C3_org(t-t3)) -> C3_org(t-t3)/1  "C3_org(t-t3)"
  fLO/1 -> Mixer E3/3(fLO)  "fLO(t)"
  Settler E3/2(C3_aq(t-t3)) -> C3_aq(t-t3)/1  "C3_aq(t-t3)"

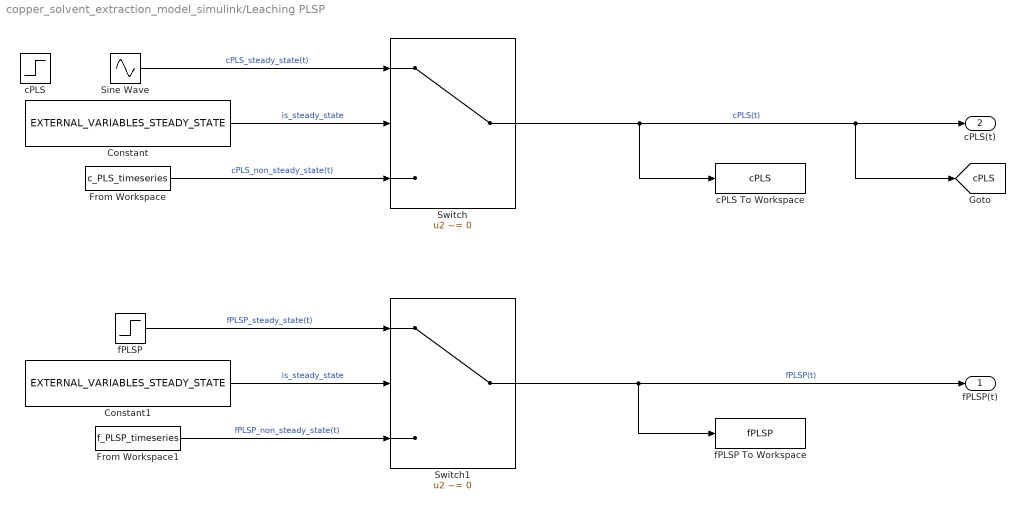
== system copper_solvent_extraction_model_simulink/Leaching PLSP ==
  Constant : Constant  Value=EXTERNAL_VARIABLES_STEADY_STATE
  Constant1 : Constant  Value=EXTERNAL_VARIABLES_STEADY_STATE
  From Workspace : FromWorkspace  VariableName=c_PLS_timeseries
  From Workspace1 : FromWorkspace  VariableName=f_PLSP_timeseries
  Sine Wave : Sin  Amplitude=1.5  Bias=7  Frequency=0.002  SampleTime=0
  Switch : Switch  Criteria=u2 ~= 0
  Switch1 : Switch  Criteria=u2 ~= 0
  cPLS : Step  Time=0  Before=cPLS_ss  After=cPLS_ss  SampleTime=0
  cPLS To Workspace : ToWorkspace  VariableName=cPLS  SaveFormat=Timeseries  SampleTime=-1
  fPLSP : Step  Time=0  Before=fPLSP_ss  After=fPLSP_ss  SampleTime=0
  fPLSP To Workspace : ToWorkspace  VariableName=fPLSP  SaveFormat=Timeseries  SampleTime=-1
  fPLSP(t) : Outport
  cPLS(t) : Outport  Port=2
  tag scope: cPLS=global
  wires:
  Switch1/1 -> fPLSP To Workspace/1, fPLSP(t)/1  "fPLSP(t)"
  Switch/1 -> cPLS To Workspace/1, [cPLS], cPLS(t)/1  "cPLS(t)"
  Constant/1 -> Switch/2  "is_steady_state"
  Constant1/1 -> Switch1/2  "is_steady_state"
  Sine Wave/1 -> Switch/1  "cPLS_steady_state(t)"
  fPLSP/1 -> Switch1/1  "fPLSP_steady_state(t)"
  From Workspace/1 -> Switch/3  "cPLS_non_steady_state(t)"
  From Workspace1/1 -> Switch1/3  "fPLSP_non_steady_state(t)"

== system copper_solvent_extraction_model_simulink/Leaching PLSS ==
  Constant1 : Constant  Value=EXTERNAL_VARIABLES_STEADY_STATE
  From Workspace : FromWorkspace  VariableName=f_PLSS_timeseries
  Switch1 : Switch  Criteria=u2 ~= 0
  fPLSS : Step  Time=0  Before=fPLSS_ss  After=fPLSS_ss  SampleTime=0
  fPLSS To Workspace : ToWorkspace  VariableName=fPLSS  SaveFormat=Timeseries  SampleTime=-1
  fPLSS(t) : Outport
  cPLS(t) : Outport  Port=2
  wires:
  [cPLS] -> cPLS(t)/1  "cPLS(t)"
  Switch1/1 -> fPLSS To Workspace/1, fPLSS(t)/1  "fPLSS(t)"
  Constant1/1 -> Switch1/2  "is_steady_state"
  fPLSS/1 -> Switch1/1  "fPLSS_steady_state(t)"
  From Workspace/1 -> Switch1/3  "fPLSS_non_steady_state(t)"

== system copper_solvent_extraction_model_simulink/Sensor c_BO ==
  c_BO(t) : Inport
  Random Number : RandomNumber  Variance=sigma_c_BO^2  Seed=seed_c_BO  SampleTime=step_time
  Sum : Sum  Inputs=++|
  To Workspace : ToWorkspace  VariableName=c_BO_measured  SaveFormat=Timeseries  SampleTime=-1
  wires:
  Sum/1 -> To Workspace/1  "c_BO_measured(t)"
  Random Number/1 -> Sum/1  "Sensor c_BO Noise"
  c_BO(t)/1 -> Sum/2  "c_BO(t)"

== system copper_solvent_extraction_model_simulink/Sensor c_LE ==
  c_LE(t) : Inport
  Random Number : RandomNumber  Variance=sigma_c_LE^2  Seed=seed_c_LE  SampleTime=step_time
  Sum : Sum  Inputs=++|
  To Workspace : ToWorkspace  VariableName=c_LE_measured  SaveFormat=Timeseries  SampleTime=-1
  c_LE_measured(t) : Outport
  tag scope: c_LE_measured=global
  wires:
  Sum/1 -> c_LE_measured(t)/1, [c_LE_measured], To Workspace/1  "c_LE_measured(t)"
  Random Number/1 -> Sum/1  "Sensor c_LE Noise"
  c_LE(t)/1 -> Sum/2  "c_LE(t)"

== system copper_solvent_extraction_model_simulink/Sensor c_LO ==
  c_LO(t) : Inport
  Random Number : RandomNumber  Variance=sigma_c_LO^2  Seed=seed_c_LO  SampleTime=step_time
  Sum : Sum  Inputs=++|
  To Workspace : ToWorkspace  VariableName=c_LO_measured  SaveFormat=Timeseries  SampleTime=-1
  c_LO_measured(t) : Outport
  tag scope: c_LO_measured=global
  wires:
  c_LO(t)/1 -> Sum/2  "c_LO(t)"
  Random Number/1 -> Sum/1  "Sensor c_LO Noise"
  Sum/1 -> c_LO_measured(t)/1, [c_LO_measured], To Workspace/1  "c_LO_measured(t)"

== system copper_solvent_extraction_model_simulink/Sensor c_PLS ==
  c_PLS(t) : Inport
  Random Number : RandomNumber  Variance=sigma_c_PLS^2  Seed=seed_c_PLS  SampleTime=step_time
  Sum : Sum  Inputs=++|
  To Workspace : ToWorkspace  VariableName=c_PLS_measured  SaveFormat=Timeseries  SampleTime=-1
  c_PLS_measured(t) : Outport
  tag scope: c_PLS_measured=global
  wires:
  c_PLS(t)/1 -> Sum/2  "c_PLS(t)"
  Random Number/1 -> Sum/1  "Sensor c_PLS Noise"
  Sum/1 -> c_PLS_measured(t)/1, [c_PLS_measured], To Workspace/1  "c_PLS_measured(t)"

== system copper_solvent_extraction_model_simulink/Sensor c_RE ==
  c_RE(t) : Inport
  Random Number : RandomNumber  Variance=sigma_c_RE^2  Seed=seed_c_RE  SampleTime=step_time
  Sum : Sum  Inputs=++|
  To Workspace : ToWorkspace  VariableName=c_RE_measured  SaveFormat=Timeseries  SampleTime=-1
  c_RE_measured(t) : Outport
  tag scope: c_RE_measured=global
  wires:
  Sum/1 -> c_RE_measured(t)/1, [c_RE_measured], To Workspace/1  "c_RE_measured(t)"
  Random Number/1 -> Sum/1  "Sensor c_RE Noise"
  c_RE(t)/1 -> Sum/2  "c_RE(t)"

== system copper_solvent_extraction_model_simulink/Sensor f_LE ==
  f_LE(t) : Inport
  Random Number : RandomNumber  Variance=sigma_f_LE^2  Seed=seed_f_LE  SampleTime=step_time
  Sum : Sum  Inputs=++|
  To Workspace : ToWorkspace  VariableName=f_LE_measured  SaveFormat=Timeseries  SampleTime=-1
  wires:
  f_LE(t)/1 -> Sum/2  "f_LE(t)"
  Random Number/1 -> Sum/1  "Sensor f_LE Noise"
  Sum/1 -> To Workspace/1  "f_LE_measured(t)"

== system copper_solvent_extraction_model_simulink/Sensor f_LO ==
  f_LO(t) : Inport
  Random Number : RandomNumber  Variance=sigma_f_LO^2  Seed=seed_f_LO  SampleTime=step_time
  Sum : Sum  Inputs=++|
  To Workspace : ToWorkspace  VariableName=f_LO_measured  SaveFormat=Timeseries  SampleTime=-1
  wires:
  Sum/1 -> To Workspace/1  "f_LO_measured(t)"
  Random Number/1 -> Sum/1  "Sensor f_LO Noise"
  f_LO(t)/1 -> Sum/2  "f_LO(t)"

== system copper_solvent_extraction_model_simulink/Sensor f_PLSP ==
  f_PLSP(t) : Inport
  Random Number : RandomNumber  Variance=sigma_f_PLSP^2  Seed=seed_f_PLSP  SampleTime=step_time
  Sum : Sum  Inputs=++|
  To Workspace : ToWorkspace  VariableName=f_PLSP_measured  SaveFormat=Timeseries  SampleTime=-1
  f_PLSP_measured(t) : Outport
  tag scope: f_PLSP_measured=global
  wires:
  Sum/1 -> f_PLSP_measured(t)/1, [f_PLSP_measured], To Workspace/1  "f_PLSP_measured(t)"
  Random Number/1 -> Sum/1  "Sensor f_PLSP noise"
  f_PLSP(t)/1 -> Sum/2  "f_PLSP(t)"

== system copper_solvent_extraction_model_simulink/Sensor f_PLSS ==
  f_PLSS(t) : Inport
  Random Number : RandomNumber  Variance=sigma_f_PLSS^2  Seed=seed_f_PLSS  SampleTime=step_time
  Sum : Sum  Inputs=++|
  To Workspace : ToWorkspace  VariableName=f_PLSS_measured  SaveFormat=Timeseries  SampleTime=-1
  f_PLSS_measured(t) : Outport
  tag scope: f_PLSS_measured=global
  wires:
  f_PLSS(t)/1 -> Sum/2  "f_PLSS(t)"
  Random Number/1 -> Sum/1  "Sensor f_PLSS Noise"
  Sum/1 -> f_PLSS_measured(t)/1, [f_PLSS_measured], To Workspace/1  "f_PLSS_measured(t)"

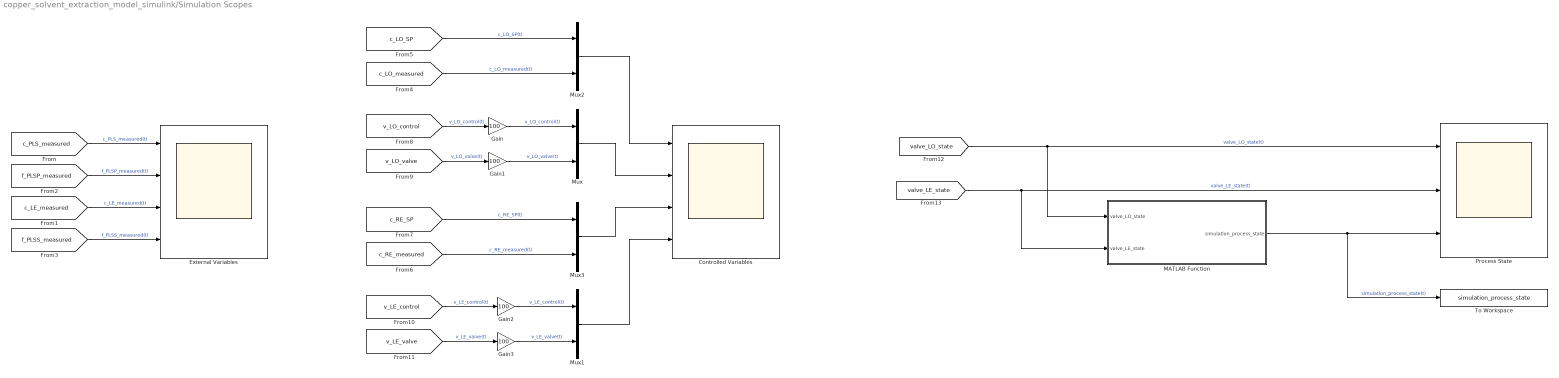
== system copper_solvent_extraction_model_simulink/Simulation Scopes ==
  Controlled Variables : Scope  NumInputPorts=4
  External Variables : Scope  NumInputPorts=4
  Gain{,1..3} (4 alike) : Gain  Gain=100
  MATLAB Function : MATLAB Function  TreatAsAtomicUnit=on
  Mux{,1..3} (4 alike) : Mux  Inputs=2
  Process State : Scope  NumInputPorts=3
  To Workspace : ToWorkspace  VariableName=simulation_process_state  SaveFormat=Timeseries  SampleTime=-1
  wires:
  [c_PLS_measured] -> External Variables/1  "c_PLS_measured(t)"
  [c_LE_measured] -> External Variables/3  "c_LE_measured(t)"
  [f_PLSP_measured] -> External Variables/2  "f_PLSP_measured(t)"
  [f_PLSS_measured] -> External Variables/4  "f_PLSS_measured(t)"
  Mux/1 -> Controlled Variables/2
  Mux1/1 -> Controlled Variables/4
  [c_LO_measured] -> Mux2/2  "c_LO_measured(t)"
  [c_LO_SP] -> Mux2/1  "c_LO_SP(t)"
  Mux2/1 -> Controlled Variables/1
  [c_RE_measured] -> Mux3/2  "c_RE_measured(t)"
  [c_RE_SP] -> Mux3/1  "c_RE_SP(t)"
  Mux3/1 -> Controlled Variables/3
  Gain/1 -> Mux/1  "v_LO_control(t)"
  [v_LO_valve] -> Gain1/1  "v_LO_valve(t)"
  [v_LE_control] -> Gain2/1  "v_LE_control(t)"
  [v_LE_valve] -> Gain3/1  "v_LE_valve(t)"
  [v_LO_control] -> Gain/1  "v_LO_control(t)"
  Gain1/1 -> Mux/2  "v_LO_valve(t)"
  Gain2/1 -> Mux1/1  "v_LE_control(t)"
  Gain3/1 -> Mux1/2  "v_LE_valve(t)"
  [valve_LO_state] -> Process State/1, MATLAB Function/1(valve_LO_state)  "valve_LO_state(t)"
  [valve_LE_state] -> Process State/2, MATLAB Function/2(valve_LE_state)  "valve_LE_state(t)"
  MATLAB Function/1(simulation_process_state) -> To Workspace/1, Process State/3  "simulation_process_state(t)"

== system copper_solvent_extraction_model_simulink/Stripping S1 ==
  C3_org(t-t3) : Inport
  fLO : Inport  Port=2
  cLE : Inport  Port=3
  fLE : Inport  Port=4
  Mixer S1 : Subsystem
      mask Display: image('.\assets\simulink\mixers_and_setlers\S1_mixer.png'); % Use "Edit Image" on toolstrip to change.
  Settler S1 : Subsystem
      mask Display: image('.\assets\simulink\mixers_and_setlers\S1_settler.png'); % Use "Edit Image" on toolstrip to change.
  C4_org(t-t4) : Outport
  fLO_out(t) : Outport  Port=2
  C1_el(t-t4) : Outport  Port=3
  wires:
  cLE/1 -> Mixer S1/2(cLE)  "cLE(t)"
  Mixer S1/2(C4_org(t)) -> Settler S1/2(C4_org(t))  "C4_org(t)"
  Mixer S1/1(C1_el(t)) -> Settler S1/1(C1_el(t))  "C1_el(t)"
  fLE/1 -> Mixer S1/1(fLE)  "fLE(t)"
  C3_org(t-t3)/1 -> Mixer S1/4(C3_org(t-t3))  "C3_org(t-t3)"
  Settler S1/1(C1_el(t-t4)) -> C1_el(t-t4)/1  "C1_el(t-t4)"
  fLO/1 -> fLO_out(t)/1, Mixer S1/3(fLO)  "fLO(t)"
  Settler S1/2(C4_org(t-t4)) -> C4_org(t-t4)/1  "C4_org(t-t4)"

== system copper_solvent_extraction_model_simulink/Valve LE ==
  vLE_control_saturated(t) : Inport
  Memory : Memory  InitialCondition=vLE_ss
  Simulation time : Clock
  Valve LE flow model : Subsystem
  Valve LE valve model : Subsystem
      settings: PortSchema="{\"entries\":[{\"content\":{\"sides\":[{\"content\":{\"connectorIds\":[\"In1\"]},\"type\":\"ConnectorPlacement.EquallySpacedRectSide\",\"uuid\":\"2e9f031d-8496-4052-a2e0-829d2345863a\"},{\"content\":{\"connectorIds\":[\"Out1\"],\"side\":\"RIGHT\"},\"type\":\"ConnectorPlacement.EquallySpacedRectSide\",\"uuid\":\"38b5eb17-cc51-4fa3-9394-ca0ed547bb78\"},{\"content\":{\"connectorIds\":[\"In2\",\"In3\",\"In4\",\"In5\"],\"side\":\"TOP\"},\"type\":\"ConnectorPlacement.EquallySpacedRectSide\",\"uuid\":\"bfeaaf73-7bd9-4ee3-b412-f379f1bcce90\"}]},\"type\":\"ConnectorPlacement.EquallySpacedConnector\",\"uuid\":\"a9e57682-026b-43fa-bec2-e5bd18169bdc\"}],\"packageUris\":[\"http://schema.mathworks.com/mf0/Connector/R2020b\"],\"version\":\"1.0\"}"
  Variant Subsystem : Subsystem  Variant=on
      mask Display: image('.\assets\simulink\valves\valve_LE_state.png'); % Use "Edit Image" on toolstrip to change.
  fLE(t) : Outport
  wires:
  Valve LE flow model/1(fLE(t)) -> fLE(t)/1  "fLE(t)"
  Variant Subsystem/1(valve_LE_state) -> Valve LE valve model/2(valve_LE_state)  "valve_LE_state(t)"
  Variant Subsystem/4(valve_LE_stiction_start_time) -> Valve LE valve model/5(valve_LE_stiction_start_time)  "valve_LE_stiction_start_time"
  Simulation time/1 -> Variant Subsystem/1(simulation_time)  "simulation_time"
  Variant Subsystem/2(v_LE_is_not_stuck) -> Valve LE valve model/3(v_LE_is_not_stuck(t))  "v_LE_is_not_stuck(t)"
  Memory/1 -> Variant Subsystem/2(v_LE_valve_previous)  "v_LE_valve_previous(t)"
  Valve LE valve model/1(v_LE_valve(t)) -> Memory/1, Valve LE flow model/1(vLE_valve(t))  "v_LE_valve(t)"
  Variant Subsystem/3(valve_LE_stiction_v_initial) -> Valve LE valve model/4(valve_LE_stiction_v_initial)  "valve_LE_stiction_v_initial"
  vLE_control_saturated(t)/1 -> Valve LE valve model/1(v_LE_control(t))  "vLE_control_saturated(t)"
